simulink model "PID_2Rotori"  (R2018b)
settings: Solver=VariableStepAuto  StartTime=0.0  StopTime=10.0  RelTol=1e-3
undefined symbols (not defined in the file): Kd, Kp, parametri, parametri_stimati
settings Model: Creator=giga4  LastModifiedBy=giga4

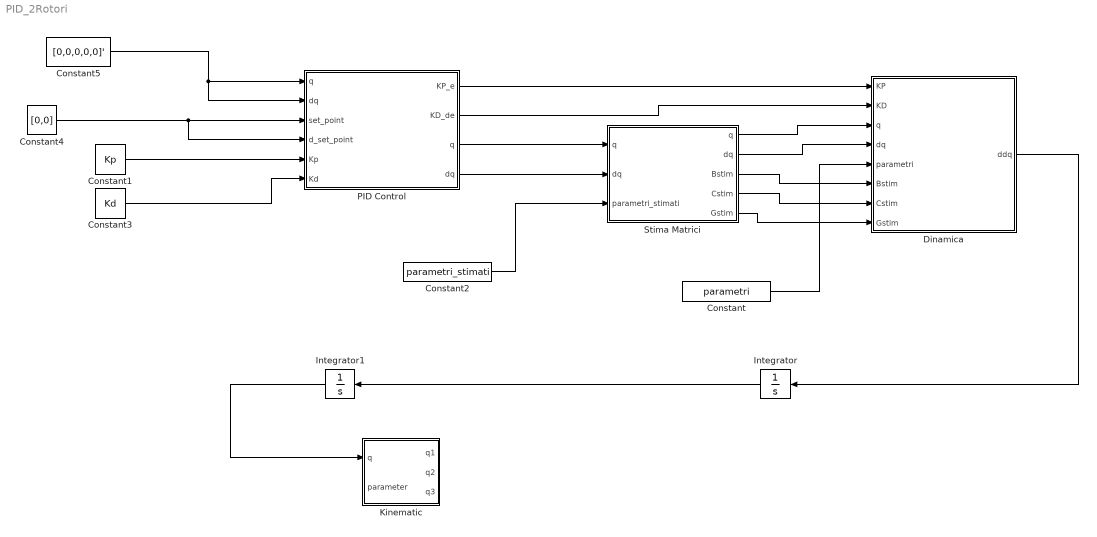
== system PID_2Rotori ==
  Constant : Constant  Value=parametri
  Constant1 : Constant  Value=Kp
  Constant2 : Constant  Value=parametri_stimati
  Constant3 : Constant  Value=Kd
  Constant4 : Constant  Value=[0,0]
  Constant5 : Constant  Value=[0,0,0,0,0]'
  Dinamica : MATLAB Function  TreatAsAtomicUnit=on
  Integrator : Integrator
  Integrator1 : Integrator
  Kinematic : MATLAB Function  TreatAsAtomicUnit=on
  PID Control : MATLAB Function  TreatAsAtomicUnit=on
  Stima Matrici : MATLAB Function  TreatAsAtomicUnit=on
  wires:
  Constant2/1 -> Stima Matrici/3(parametri_stimati)
  PID Control/4(dq) -> Stima Matrici/2("dq ")
  PID Control/3(q) -> Stima Matrici/1("q ")
  Dinamica/1(ddq) -> Integrator/1
  Integrator/1 -> Integrator1/1
  Constant1/1 -> PID Control/5(Kp)
  Constant3/1 -> PID Control/6(Kd)
  Constant4/1 -> PID Control/4(d_set_point), PID Control/3(set_point)
  Constant5/1 -> PID Control/2("dq "), PID Control/1("q ")
  PID Control/1(KP_e) -> Dinamica/1(KP)
  PID Control/2(KD_de) -> Dinamica/2(KD)
  Stima Matrici/1(q) -> Dinamica/3(q)
  Stima Matrici/2(dq) -> Dinamica/4(dq)
  Constant/1 -> Dinamica/5(parametri)
  Stima Matrici/3(Bstim) -> Dinamica/6(Bstim)
  Stima Matrici/4(Cstim) -> Dinamica/7(Cstim)
  Stima Matrici/5(Gstim) -> Dinamica/8(Gstim)
  Integrator1/1 -> Kinematic/1(q)

== matlab function PID_2Rotori/PID Control ==
  data: KP_e output; q input; dq input; set_point input; KD_de output; d_set_point input; Kp input; Kd input; q output; dq output
function [KP_e,KD_de,q,dq] = Control(q,dq,set_point,d_set_point,Kp,Kd) 
    e = zeros(5,1);
    de = zeros(5,1);
   
    
    e(4) = q(1)-set_point(1);
    e(5) = q(2)-set_point(2);
    de(4) = dq(1)-d_set_point(1);
    de(5) = dq(2)-d_set_point(2);
        
    M1 = [0,0,0,0,0;
          0,0,0,0,0;
          0,0,0,0,0;
          0,0,0,1,0;
          0,0,0,0,1];
    
    KD_de = M1*Kd*de;
    KP_e = M1*Kp*e;
end

== matlab function PID_2Rotori/Kinematic ==
  data: q input; q1 output; q2 output; q3 output; parameter input
function [q1,q2,q3] = Kinematic(q,parameter)

x1 = q(1);
x2 = q(2);
x3 = q(3);

L = parameter(4);

R = Rx_rad(x1)*Ry_rad(x2)*Rz_rad(x3);

T = [R, R*[0,0,L]';
     0,0,0,1];

q1 = T(1,4);
q2 = T(2,4);
q3 = T(3,4);

end

== matlab function PID_2Rotori/Stima Matrici ==
  data: q output; dq output; q input; Bstim output; Cstim output; Gstim output; dq input; parametri_stimati input
function [q,dq,Bstim,Cstim,Gstim]  = Matrici_stimate(q,dq,parametri_stimati)

    Bstim = gen_dinamica_B(q,parametri_stimati);
    Cstim = gen_dinamica_C(q,dq,parametri_stimati);
    Gstim = gen_dinamica_G(q,parametri_stimati);
    
end

== matlab function PID_2Rotori/Dinamica ==
  data: KP input; KD input; q input; ddq output; dq input; parametri input; Bstim input; Cstim input; Gstim input
function ddq = Dinamica(KP,KD,q,dq,parametri,Bstim,Cstim,Gstim)

    B = gen_dinamica_B(q,parametri);
    C = gen_dinamica_C(q,dq,parametri);
    G = gen_dinamica_G(q,parametri);
    
    ddq = B\(KD+KP-C*dq+Gstim-G);

end
